simulink model "Cascata_un_anello_2019"  (R2019b)
settings: Solver=VariableStepAuto  StartTime=0.0  StopTime=4  RelTol=1e-3
values from neighbouring files (symbols this model uses):
  den_mag_C = Gden{1}    [Controllo_un_anello_v2.m]    (also in controllo_un_anello.m)
  den_mag_C2 = Gden{1}    [Controllo_un_anello_v2.m]    (also in Controllore_testato.m; controllo_un_anello.m)
  den_mag_C3 = Gden{1}    [Controllo_un_anello_v2.m]    (also in controllo_un_anello.m)
  den_mag_M = Gden{1}    [Controllo_un_anello_v2.m]    (also in Controllore_testato.m; controllo_un_anello.m)
  Lower_bound_V = -23    [Controllo_un_anello_v2.m]    (also in Controllore_testato.m = 0; controllo_un_anello.m; controllore_piu_anelli.m)
  num_mag_C = Gnum{1}    [Controllo_un_anello_v2.m]    (also in controllo_un_anello.m)
  num_mag_C2 = Gnum{1}    [Controllo_un_anello_v2.m]    (also in Controllore_testato.m; controllo_un_anello.m)
  num_mag_C3 = Gnum{1}    [Controllo_un_anello_v2.m]    (also in controllo_un_anello.m)
  num_mag_M = Gnum{1}    [Controllo_un_anello_v2.m]    (also in Controllore_testato.m; controllo_un_anello.m)
  ueq = 15/Rtot    [controllore_piu_anelli.m]
  Upper_bound_V = 23    [Controllo_un_anello_v2.m]    (also in Controllore_testato.m; controllo_un_anello.m; controllore_piu_anelli.m)
  Veq = 12    [controllo_un_anello.m]
  x1_eq = 0.0044    [Controllo_un_anello_v2.m]    (also in Controllore_testato.m)
undefined symbols (not defined in the file or in its folder): ki, ki2, ki3, kp, kp2, kp3, Lc, Rtot, y0
libraries: simulink x6, SignalEditorBlockLib x1
settings Model: Creator=lollo  LastModifiedBy=lollo
settings DebuggingCC: UnconnectedInputMsg=none  UnconnectedOutputMsg=none  UnconnectedLineMsg=none
settings ModelReferenceCC: EnableRefExpFcnMdlSchedulingChecks=off
settings RTWCC: Description=Generic Real-Time Target

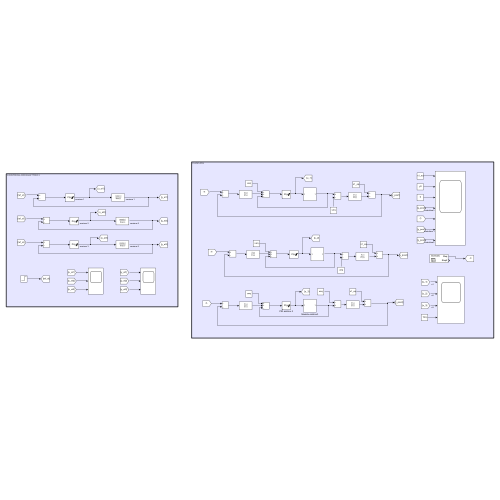
[thumbnail: Simulink's stored preview of the top-level diagram]
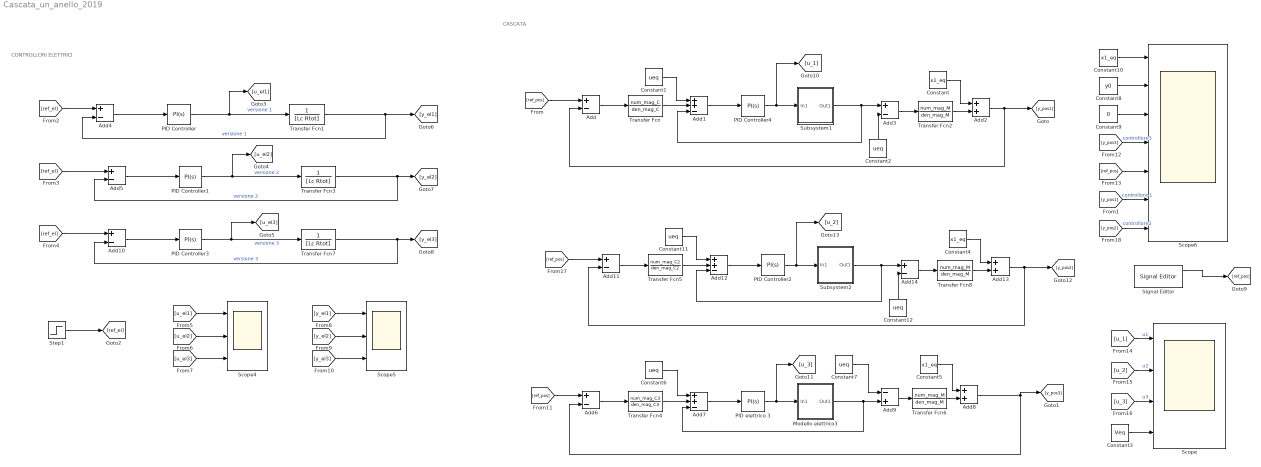
== system Cascata_un_anello_2019 ==
  note: CASCATA
  note: CONTROLLORI ELETTRICI
  Add{,3..6,10..11,14} (8 alike) : Sum  Inputs=+-
  Add1 : Sum  Inputs=++-
  Add12 : Sum  Inputs=++-
  Add13 : Sum
  Add2 : Sum
  Add7 : Sum  Inputs=++-
  Add8 : Sum
  Add9 : Sum  Inputs=-+
  Constant{,4..5,10} (4 alike) : Constant  Value=x1_eq
  Constant{1..2,6..7,11..12} (6 alike) : Constant  Value=ueq
  Constant3 : Constant  Value=Veq
  Constant8 : Constant  Value=y0
  Constant9 : Constant  Value=0
  Modello elettrico3 : Subsystem
  PID Controller : simulink/Continuous/PID Controller  Controller=PI  Form=Parallel  TimeDomain=Continuous-time  SampleTime=-1  IntegratorMethod=Forward Euler  FilterMethod=Forward Euler  ControllerParametersSource=internal  P=kp  I=ki  D=0  N=100  UseFilter=on  TunerSelectOption=Transfer Function Based (PID Tuner App)  InitialConditionSource=internal  InitialConditionForIntegrator=0  InitialConditionForFilter=0  DifferentiatorICPrevScaledInput=0  ExternalReset=none  TrackingMode=off  Kt=1  LimitOutput=on  UpperSaturationLimit=23  LowerSaturationLimit=-23  LinearizeAsGain=on  AntiWindupMode=none  Kb=1  POutMin=[]  POutMax=[]  IOutMin=[]  IOutMax=[]  DOutMin=[]  DOutMax=[]  NOutMin=[]  NOutMax=[]  SumOutMin=[]  SumOutMax=[]  SaturationOutMin=[]  SaturationOutMax=[]  PParamMin=[]  PParamMax=[]  IParamMin=[]  IParamMax=[]  DParamMin=[]  DParamMax=[]  NParamMin=[]  NParamMax=[]  KbParamMin=[]  KbParamMax=[]  KtParamMin=[]  KtParamMax=[]  KbOutMin=[]  KbOutMax=[]  KtOutMin=[]  KtOutMax=[]  IntegratorOutMin=[]  IntegratorOutMax=[]  FilterOutMin=[]  FilterOutMax=[]  SumI1OutMin=[]  SumI1OutMax=[]  SumI2OutMin=[]  SumI2OutMax=[]  SumI3OutMin=[]  SumI3OutMax=[]  SumI4OutMin=[]  SumI4OutMax=[]  SumDOutMin=[]  SumDOutMax=[]  DifferentiatorOutMin=[]  DifferentiatorOutMax=[]  FilterDiffOutCoefMin=[]  FilterDiffOutCoefMax=[]  ReciprocalOutMin=[]  ReciprocalOutMax=[]  SumDenOutMin=[]  SumDenOutMax=[]  SumNumOutMin=[]  SumNumOutMax=[]  DivideOutMin=[]  DivideOutMax=[]  IntegratorContinuousStateAttributes=''  IntegratorStateMustResolveToSignalObject=off  IntegratorRTWStateStorageClass=Auto  FilterContinuousStateAttributes=''  FilterStateMustResolveToSignalObject=off  FilterRTWStateStorageClass=Auto  ParallelPVariant=InternalParameters  IdealPVariant=Disabled  IVariant=InternalParameters  DVariant=Disabled  IntegratorVariant=Continuous  SatVariant=Enabled  AWVariant=Passthrough  PCopyVariant=Disabled  TRVariant=Disabled  FdbkBlocksVariant=Forward  IdealPFdbkVariant=Disabled  SatFdbkVariant=Disabled  DerivativeFilterVariant=Disabled  NVariant=Disabled  NCopyVariant=Disabled_SignalSpec  FilterICVariant=Disabled  IntegratorICVariant=InternalICs  ExternalResetVariant=Disabled  TRSumVariant=Passthrough  SumFdbkVariant=Disabled  SumVariant=Sum_PI
  PID Controller1 : simulink/Continuous/PID Controller  Controller=PI  Form=Parallel  TimeDomain=Continuous-time  SampleTime=-1  IntegratorMethod=Forward Euler  FilterMethod=Forward Euler  ControllerParametersSource=internal  P=kp2  I=ki2  D=0  N=100  UseFilter=on  TunerSelectOption=Transfer Function Based (PID Tuner App)  InitialConditionSource=internal  InitialConditionForIntegrator=0  InitialConditionForFilter=0  DifferentiatorICPrevScaledInput=0  ExternalReset=none  TrackingMode=off  Kt=1  LimitOutput=on  UpperSaturationLimit=23  LowerSaturationLimit=-23  LinearizeAsGain=on  AntiWindupMode=none  Kb=1  POutMin=[]  POutMax=[]  IOutMin=[]  IOutMax=[]  DOutMin=[]  DOutMax=[]  NOutMin=[]  NOutMax=[]  SumOutMin=[]  SumOutMax=[]  SaturationOutMin=[]  SaturationOutMax=[]  PParamMin=[]  PParamMax=[]  IParamMin=[]  IParamMax=[]  DParamMin=[]  DParamMax=[]  NParamMin=[]  NParamMax=[]  KbParamMin=[]  KbParamMax=[]  KtParamMin=[]  KtParamMax=[]  KbOutMin=[]  KbOutMax=[]  KtOutMin=[]  KtOutMax=[]  IntegratorOutMin=[]  IntegratorOutMax=[]  FilterOutMin=[]  FilterOutMax=[]  SumI1OutMin=[]  SumI1OutMax=[]  SumI2OutMin=[]  SumI2OutMax=[]  SumI3OutMin=[]  SumI3OutMax=[]  SumI4OutMin=[]  SumI4OutMax=[]  SumDOutMin=[]  SumDOutMax=[]  DifferentiatorOutMin=[]  DifferentiatorOutMax=[]  FilterDiffOutCoefMin=[]  FilterDiffOutCoefMax=[]  ReciprocalOutMin=[]  ReciprocalOutMax=[]  SumDenOutMin=[]  SumDenOutMax=[]  SumNumOutMin=[]  SumNumOutMax=[]  DivideOutMin=[]  DivideOutMax=[]  IntegratorContinuousStateAttributes=''  IntegratorStateMustResolveToSignalObject=off  IntegratorRTWStateStorageClass=Auto  FilterContinuousStateAttributes=''  FilterStateMustResolveToSignalObject=off  FilterRTWStateStorageClass=Auto  ParallelPVariant=InternalParameters  IdealPVariant=Disabled  IVariant=InternalParameters  DVariant=Disabled  IntegratorVariant=Continuous  SatVariant=Enabled  AWVariant=Passthrough  PCopyVariant=Disabled  TRVariant=Disabled  FdbkBlocksVariant=Forward  IdealPFdbkVariant=Disabled  SatFdbkVariant=Disabled  DerivativeFilterVariant=Disabled  NVariant=Disabled  NCopyVariant=Disabled_SignalSpec  FilterICVariant=Disabled  IntegratorICVariant=InternalICs  ExternalResetVariant=Disabled  TRSumVariant=Passthrough  SumFdbkVariant=Disabled  SumVariant=Sum_PI
  PID Controller2 : simulink/Continuous/PID Controller  Controller=PI  Form=Parallel  TimeDomain=Continuous-time  SampleTime=-1  IntegratorMethod=Forward Euler  FilterMethod=Forward Euler  ControllerParametersSource=internal  P=kp2  I=ki2  D=0  N=100  UseFilter=on  TunerSelectOption=Transfer Function Based (PID Tuner App)  InitialConditionSource=internal  InitialConditionForIntegrator=Veq  InitialConditionForFilter=0  DifferentiatorICPrevScaledInput=0  ExternalReset=none  TrackingMode=off  Kt=1  LimitOutput=on  UpperSaturationLimit=Upper_bound_V  LowerSaturationLimit=Lower_bound_V  LinearizeAsGain=on  AntiWindupMode=clamping  Kb=1  POutMin=[]  POutMax=[]  IOutMin=[]  IOutMax=[]  DOutMin=[]  DOutMax=[]  NOutMin=[]  NOutMax=[]  SumOutMin=[]  SumOutMax=[]  SaturationOutMin=[]  SaturationOutMax=[]  PParamMin=[]  PParamMax=[]  IParamMin=[]  IParamMax=[]  DParamMin=[]  DParamMax=[]  NParamMin=[]  NParamMax=[]  KbParamMin=[]  KbParamMax=[]  KtParamMin=[]  KtParamMax=[]  KbOutMin=[]  KbOutMax=[]  KtOutMin=[]  KtOutMax=[]  IntegratorOutMin=[]  IntegratorOutMax=[]  FilterOutMin=[]  FilterOutMax=[]  SumI1OutMin=[]  SumI1OutMax=[]  SumI2OutMin=[]  SumI2OutMax=[]  SumI3OutMin=[]  SumI3OutMax=[]  SumI4OutMin=[]  SumI4OutMax=[]  SumDOutMin=[]  SumDOutMax=[]  DifferentiatorOutMin=[]  DifferentiatorOutMax=[]  FilterDiffOutCoefMin=[]  FilterDiffOutCoefMax=[]  ReciprocalOutMin=[]  ReciprocalOutMax=[]  SumDenOutMin=[]  SumDenOutMax=[]  SumNumOutMin=[]  SumNumOutMax=[]  DivideOutMin=[]  DivideOutMax=[]  IntegratorContinuousStateAttributes=''  IntegratorStateMustResolveToSignalObject=off  IntegratorRTWStateStorageClass=Auto  FilterContinuousStateAttributes=''  FilterStateMustResolveToSignalObject=off  FilterRTWStateStorageClass=Auto  ParallelPVariant=InternalParameters  IdealPVariant=Disabled  IVariant=InternalParameters  DVariant=Disabled  IntegratorVariant=Continuous  SatVariant=Enabled  AWVariant=ContClampingParallel  PCopyVariant=Disabled  TRVariant=Disabled  FdbkBlocksVariant=Forward  IdealPFdbkVariant=Disabled  SatFdbkVariant=Disabled  DerivativeFilterVariant=Disabled  NVariant=Disabled  NCopyVariant=Disabled_SignalSpec  FilterICVariant=Disabled  IntegratorICVariant=InternalICs  ExternalResetVariant=Disabled  TRSumVariant=Passthrough  SumFdbkVariant=Disabled  SumVariant=Sum_PI
  PID Controller3 : simulink/Continuous/PID Controller  Controller=PI  Form=Parallel  TimeDomain=Continuous-time  SampleTime=-1  IntegratorMethod=Forward Euler  FilterMethod=Forward Euler  ControllerParametersSource=internal  P=kp3  I=ki3  D=0  N=100  UseFilter=on  TunerSelectOption=Transfer Function Based (PID Tuner App)  InitialConditionSource=internal  InitialConditionForIntegrator=0  InitialConditionForFilter=0  DifferentiatorICPrevScaledInput=0  ExternalReset=none  TrackingMode=off  Kt=1  LimitOutput=on  UpperSaturationLimit=23  LowerSaturationLimit=-23  LinearizeAsGain=on  AntiWindupMode=none  Kb=1  POutMin=[]  POutMax=[]  IOutMin=[]  IOutMax=[]  DOutMin=[]  DOutMax=[]  NOutMin=[]  NOutMax=[]  SumOutMin=[]  SumOutMax=[]  SaturationOutMin=[]  SaturationOutMax=[]  PParamMin=[]  PParamMax=[]  IParamMin=[]  IParamMax=[]  DParamMin=[]  DParamMax=[]  NParamMin=[]  NParamMax=[]  KbParamMin=[]  KbParamMax=[]  KtParamMin=[]  KtParamMax=[]  KbOutMin=[]  KbOutMax=[]  KtOutMin=[]  KtOutMax=[]  IntegratorOutMin=[]  IntegratorOutMax=[]  FilterOutMin=[]  FilterOutMax=[]  SumI1OutMin=[]  SumI1OutMax=[]  SumI2OutMin=[]  SumI2OutMax=[]  SumI3OutMin=[]  SumI3OutMax=[]  SumI4OutMin=[]  SumI4OutMax=[]  SumDOutMin=[]  SumDOutMax=[]  DifferentiatorOutMin=[]  DifferentiatorOutMax=[]  FilterDiffOutCoefMin=[]  FilterDiffOutCoefMax=[]  ReciprocalOutMin=[]  ReciprocalOutMax=[]  SumDenOutMin=[]  SumDenOutMax=[]  SumNumOutMin=[]  SumNumOutMax=[]  DivideOutMin=[]  DivideOutMax=[]  IntegratorContinuousStateAttributes=''  IntegratorStateMustResolveToSignalObject=off  IntegratorRTWStateStorageClass=Auto  FilterContinuousStateAttributes=''  FilterStateMustResolveToSignalObject=off  FilterRTWStateStorageClass=Auto  ParallelPVariant=InternalParameters  IdealPVariant=Disabled  IVariant=InternalParameters  DVariant=Disabled  IntegratorVariant=Continuous  SatVariant=Enabled  AWVariant=Passthrough  PCopyVariant=Disabled  TRVariant=Disabled  FdbkBlocksVariant=Forward  IdealPFdbkVariant=Disabled  SatFdbkVariant=Disabled  DerivativeFilterVariant=Disabled  NVariant=Disabled  NCopyVariant=Disabled_SignalSpec  FilterICVariant=Disabled  IntegratorICVariant=InternalICs  ExternalResetVariant=Disabled  TRSumVariant=Passthrough  SumFdbkVariant=Disabled  SumVariant=Sum_PI
  PID Controller4 : simulink/Continuous/PID Controller  Controller=PI  Form=Parallel  TimeDomain=Continuous-time  SampleTime=-1  IntegratorMethod=Forward Euler  FilterMethod=Forward Euler  ControllerParametersSource=internal  P=kp  I=ki  D=0  N=100  UseFilter=on  TunerSelectOption=Transfer Function Based (PID Tuner App)  InitialConditionSource=internal  InitialConditionForIntegrator=Veq  InitialConditionForFilter=0  DifferentiatorICPrevScaledInput=0  ExternalReset=none  TrackingMode=off  Kt=1  LimitOutput=on  UpperSaturationLimit=Upper_bound_V  LowerSaturationLimit=Lower_bound_V  LinearizeAsGain=on  AntiWindupMode=clamping  Kb=1  POutMin=[]  POutMax=[]  IOutMin=[]  IOutMax=[]  DOutMin=[]  DOutMax=[]  NOutMin=[]  NOutMax=[]  SumOutMin=[]  SumOutMax=[]  SaturationOutMin=[]  SaturationOutMax=[]  PParamMin=[]  PParamMax=[]  IParamMin=[]  IParamMax=[]  DParamMin=[]  DParamMax=[]  NParamMin=[]  NParamMax=[]  KbParamMin=[]  KbParamMax=[]  KtParamMin=[]  KtParamMax=[]  KbOutMin=[]  KbOutMax=[]  KtOutMin=[]  KtOutMax=[]  IntegratorOutMin=[]  IntegratorOutMax=[]  FilterOutMin=[]  FilterOutMax=[]  SumI1OutMin=[]  SumI1OutMax=[]  SumI2OutMin=[]  SumI2OutMax=[]  SumI3OutMin=[]  SumI3OutMax=[]  SumI4OutMin=[]  SumI4OutMax=[]  SumDOutMin=[]  SumDOutMax=[]  DifferentiatorOutMin=[]  DifferentiatorOutMax=[]  FilterDiffOutCoefMin=[]  FilterDiffOutCoefMax=[]  ReciprocalOutMin=[]  ReciprocalOutMax=[]  SumDenOutMin=[]  SumDenOutMax=[]  SumNumOutMin=[]  SumNumOutMax=[]  DivideOutMin=[]  DivideOutMax=[]  IntegratorContinuousStateAttributes=''  IntegratorStateMustResolveToSignalObject=off  IntegratorRTWStateStorageClass=Auto  FilterContinuousStateAttributes=''  FilterStateMustResolveToSignalObject=off  FilterRTWStateStorageClass=Auto  ParallelPVariant=InternalParameters  IdealPVariant=Disabled  IVariant=InternalParameters  DVariant=Disabled  IntegratorVariant=Continuous  SatVariant=Enabled  AWVariant=ContClampingParallel  PCopyVariant=Disabled  TRVariant=Disabled  FdbkBlocksVariant=Forward  IdealPFdbkVariant=Disabled  SatFdbkVariant=Disabled  DerivativeFilterVariant=Disabled  NVariant=Disabled  NCopyVariant=Disabled_SignalSpec  FilterICVariant=Disabled  IntegratorICVariant=InternalICs  ExternalResetVariant=Disabled  TRSumVariant=Passthrough  SumFdbkVariant=Disabled  SumVariant=Sum_PI
  PID elettrico 3 : simulink/Continuous/PID Controller  Controller=PI  Form=Parallel  TimeDomain=Continuous-time  SampleTime=-1  IntegratorMethod=Forward Euler  FilterMethod=Forward Euler  ControllerParametersSource=internal  P=kp3  I=ki3  D=0  N=100  UseFilter=on  TunerSelectOption=Transfer Function Based (PID Tuner App)  InitialConditionSource=internal  InitialConditionForIntegrator=Veq  InitialConditionForFilter=0  DifferentiatorICPrevScaledInput=0  ExternalReset=none  TrackingMode=off  Kt=1  LimitOutput=on  UpperSaturationLimit=Upper_bound_V  LowerSaturationLimit=Lower_bound_V  LinearizeAsGain=on  AntiWindupMode=none  Kb=1  POutMin=[]  POutMax=[]  IOutMin=[]  IOutMax=[]  DOutMin=[]  DOutMax=[]  NOutMin=[]  NOutMax=[]  SumOutMin=[]  SumOutMax=[]  SaturationOutMin=[]  SaturationOutMax=[]  PParamMin=[]  PParamMax=[]  IParamMin=[]  IParamMax=[]  DParamMin=[]  DParamMax=[]  NParamMin=[]  NParamMax=[]  KbParamMin=[]  KbParamMax=[]  KtParamMin=[]  KtParamMax=[]  KbOutMin=[]  KbOutMax=[]  KtOutMin=[]  KtOutMax=[]  IntegratorOutMin=[]  IntegratorOutMax=[]  FilterOutMin=[]  FilterOutMax=[]  SumI1OutMin=[]  SumI1OutMax=[]  SumI2OutMin=[]  SumI2OutMax=[]  SumI3OutMin=[]  SumI3OutMax=[]  SumI4OutMin=[]  SumI4OutMax=[]  SumDOutMin=[]  SumDOutMax=[]  DifferentiatorOutMin=[]  DifferentiatorOutMax=[]  FilterDiffOutCoefMin=[]  FilterDiffOutCoefMax=[]  ReciprocalOutMin=[]  ReciprocalOutMax=[]  SumDenOutMin=[]  SumDenOutMax=[]  SumNumOutMin=[]  SumNumOutMax=[]  DivideOutMin=[]  DivideOutMax=[]  IntegratorContinuousStateAttributes=''  IntegratorStateMustResolveToSignalObject=off  IntegratorRTWStateStorageClass=Auto  FilterContinuousStateAttributes=''  FilterStateMustResolveToSignalObject=off  FilterRTWStateStorageClass=Auto  ParallelPVariant=InternalParameters  IdealPVariant=Disabled  IVariant=InternalParameters  DVariant=Disabled  IntegratorVariant=Continuous  SatVariant=Enabled  AWVariant=Passthrough  PCopyVariant=Disabled  TRVariant=Disabled  FdbkBlocksVariant=Forward  IdealPFdbkVariant=Disabled  SatFdbkVariant=Disabled  DerivativeFilterVariant=Disabled  NVariant=Disabled  NCopyVariant=Disabled_SignalSpec  FilterICVariant=Disabled  IntegratorICVariant=InternalICs  ExternalResetVariant=Disabled  TRSumVariant=Passthrough  SumFdbkVariant=Disabled  SumVariant=Sum_PI
  Scope : Scope  NumInputPorts=4
  Scope4 : Scope  NumInputPorts=3
  Scope5 : Scope  NumInputPorts=3
  Scope6 : Scope  NumInputPorts=7
  Signal Editor : SignalEditorBlockLib/Signal Editor  FileName=input_signal.mat  ActiveScenario=Scenario  ActiveSignal=Step  IsBus=off  OutputBusObjectStr=Bus: BusObject  SampleTime=0  Interpolate=off  ZeroCross=off  OutputAfterFinalValue=Setting to zero  Unit=inherit  PreserveSignalName=on
  Step1 : Step  After=Vref/Rtot  SampleTime=0
  Subsystem1 : Subsystem
  Subsystem2 : Subsystem
  Transfer Fcn : TransferFcn  Numerator=num_mag_C  Denominator=den_mag_C
  Transfer Fcn1 : TransferFcn  Denominator=[Lc Rtot]
  Transfer Fcn2 : TransferFcn  Numerator=num_mag_M  Denominator=den_mag_M
  Transfer Fcn3 : TransferFcn  Denominator=[Lc Rtot]
  Transfer Fcn4 : TransferFcn  Numerator=num_mag_C3  Denominator=den_mag_C3
  Transfer Fcn5 : TransferFcn  Numerator=num_mag_C2  Denominator=den_mag_C2
  Transfer Fcn6 : TransferFcn  Numerator=num_mag_M  Denominator=den_mag_M
  Transfer Fcn7 : TransferFcn  Denominator=[Lc Rtot]
  Transfer Fcn8 : TransferFcn  Numerator=num_mag_M  Denominator=den_mag_M
  wires:
  Add/1 -> Transfer Fcn/1
  Transfer Fcn/1 -> Add1/2
  [ref_pos] -> Add/1
  Transfer Fcn2/1 -> Add2/2
  Constant/1 -> Add2/1
  Add2/1 -> Add/2, [y_pos1]
  Add3/1 -> Transfer Fcn2/1
  Constant2/1 -> Add3/2
  PID Controller4/1 -> [u_1], Subsystem1/1(In1)
  Add1/1 -> PID Controller4/1
  Subsystem1/1(Out1) -> Add1/3, Add3/1
  Transfer Fcn1/1 -> [y_el1], Add4/2  "versione 1"
  Add4/1 -> PID Controller/1
  PID Controller/1 -> [u_el1], Transfer Fcn1/1  "versione 1"
  Transfer Fcn3/1 -> Add5/2, [y_el2]  "versione 2"
  Add5/1 -> PID Controller1/1
  PID Controller1/1 -> [u_el2], Transfer Fcn3/1  "versione 2"
  Add6/1 -> Transfer Fcn4/1
  Transfer Fcn4/1 -> Add7/2
  Add7/1 -> PID elettrico 3/1
  Modello elettrico3/1(Out1) -> Add9/2, Add7/3
  PID elettrico 3/1 -> [u_3], Modello elettrico3/1(In1)
  Transfer Fcn6/1 -> Add8/2
  Add9/1 -> Transfer Fcn6/1
  Add8/1 -> [y_pos3], Add6/2
  Constant5/1 -> Add8/1
  Constant7/1 -> Add9/1
  Constant6/1 -> Add7/1
  Constant1/1 -> Add1/1
  Step1/1 -> [ref_el]
  [ref_el] -> Add4/1
  [ref_el] -> Add5/1
  [ref_el] -> Add10/1
  Transfer Fcn7/1 -> [y_el3], Add10/2  "versione 3"
  PID Controller3/1 -> [u_el3], Transfer Fcn7/1  "versione 3"
  Add10/1 -> PID Controller3/1
  [u_el1] -> Scope4/1
  [u_el2] -> Scope4/2
  [u_el3] -> Scope4/3
  [y_el2] -> Scope5/2
  [y_el3] -> Scope5/3
  [y_el1] -> Scope5/1
  Signal Editor/1 -> [ref_pos]
  [ref_pos] -> Add6/1
  [y_pos3] -> Scope6/4  "controllore3"
  [ref_pos] -> Scope6/5
  Constant8/1 -> Scope6/2
  Constant9/1 -> Scope6/3
  Constant10/1 -> Scope6/1
  [y_pos1] -> Scope6/6  "controllore 1"
  [u_1] -> Scope/1  "u1"
  [u_2] -> Scope/2  "u2"
  [u_3] -> Scope/3  "u3"
  Constant3/1 -> Scope/4
  PID Controller2/1 -> [u_2], Subsystem2/1(In1)
  Constant11/1 -> Add12/1
  Constant4/1 -> Add13/1
  [ref_pos] -> Add11/1
  Transfer Fcn5/1 -> Add12/2
  Subsystem2/1(Out1) -> Add12/3, Add14/1
  Add11/1 -> Transfer Fcn5/1
  Add12/1 -> PID Controller2/1
  Add14/1 -> Transfer Fcn8/1
  Constant12/1 -> Add14/2
  Transfer Fcn8/1 -> Add13/2
  Add13/1 -> Add11/2, [y_pos2]
  [y_pos2] -> Scope6/7  "controllore2"

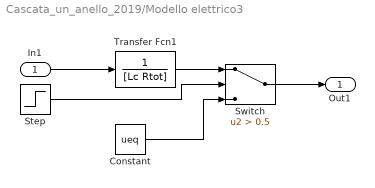
== system Cascata_un_anello_2019/Modello elettrico3 ==
  In1 : Inport
  Constant : Constant  Value=ueq
  Step : Step  Time=0.5  SampleTime=0
  Switch : Switch  Criteria=u2 > Threshold  Threshold=0.5
  Transfer Fcn1 : TransferFcn  Denominator=[Lc Rtot]
  Out1 : Outport
  wires:
  Transfer Fcn1/1 -> Switch/1
  In1/1 -> Transfer Fcn1/1
  Switch/1 -> Out1/1
  Step/1 -> Switch/2
  Constant/1 -> Switch/3

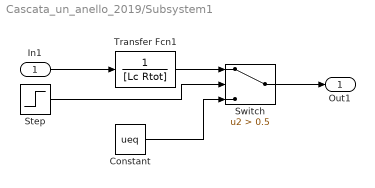
== system Cascata_un_anello_2019/Subsystem1 ==
  In1 : Inport
  Constant : Constant  Value=ueq
  Step : Step  Time=0.5  SampleTime=0
  Switch : Switch  Criteria=u2 > Threshold  Threshold=0.5
  Transfer Fcn1 : TransferFcn  Denominator=[Lc Rtot]
  Out1 : Outport
  wires:
  Transfer Fcn1/1 -> Switch/1
  In1/1 -> Transfer Fcn1/1
  Switch/1 -> Out1/1
  Step/1 -> Switch/2
  Constant/1 -> Switch/3

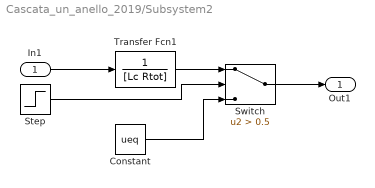
== system Cascata_un_anello_2019/Subsystem2 ==
  In1 : Inport
  Constant : Constant  Value=ueq
  Step : Step  Time=0.5  SampleTime=0
  Switch : Switch  Criteria=u2 > Threshold  Threshold=0.5
  Transfer Fcn1 : TransferFcn  Denominator=[Lc Rtot]
  Out1 : Outport
  wires:
  Transfer Fcn1/1 -> Switch/1
  In1/1 -> Transfer Fcn1/1
  Switch/1 -> Out1/1
  Step/1 -> Switch/2
  Constant/1 -> Switch/3
